simulink model "observer"  (R2023b)
settings: Solver=VariableStepAuto  StartTime=0.0  StopTime=10.0  FixedStep=0.0066666666666666671  MaxStep=0.1e-3
undefined symbols (not defined in the file or in its folder): A_obs, AMPLITUDE, B_obs, C_obs, D_obs, FREQUENCY
settings Model: Creator=gosmann  LastModifiedBy=gosmann
settings SolverCC: MaxConsecutiveMinStep=100

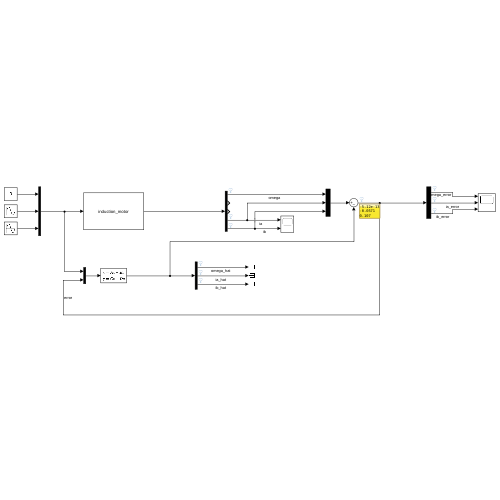
[thumbnail: Simulink's stored preview of the top-level diagram]
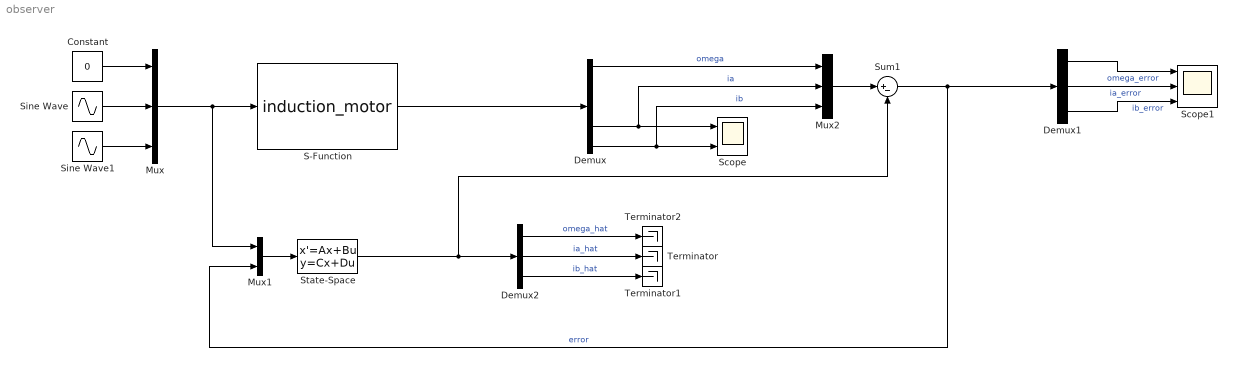
== system observer ==
  Constant : Constant  Value=0
  Demux : Demux  Outputs=5
  Demux1 : Demux  Outputs=3
  Demux2 : Demux  Outputs=3
  Mux : Mux  Inputs=3
  Mux1 : Mux  Inputs=2
  Mux2 : Mux  Inputs=3
  S-Function : S-Function  FunctionName=induction_motor  Parameters=parameters  SFunctionDeploymentMode=off  EnableBusSupport=off
  Scope : Scope  NumInputPorts=2
  Scope1 : Scope  NumInputPorts=3
  Sine Wave : Sin  Amplitude=AMPLITUDE  Frequency=FREQUENCY  SampleTime=0
  Sine Wave1 : Sin  Amplitude=AMPLITUDE  Frequency=FREQUENCY  Phase=0-(pi/180)*90  SampleTime=0
  State-Space : StateSpace  A=A_obs  B=B_obs  C=C_obs  D=D_obs  InitialCondition=[ 0 0 0 0 0 ]
  Sum1 : Sum  Inputs=|+-
  Terminator : Terminator
  Terminator1 : Terminator
  Terminator2 : Terminator
  wires:
  S-Function/1 -> Demux/1
  Mux/1 -> Mux1/1, S-Function/1
  Sine Wave1/1 -> Mux/3
  Sine Wave/1 -> Mux/2
  Constant/1 -> Mux/1
  Demux/4 -> Mux2/2, Scope/1  "ia"
  Demux/5 -> Mux2/3, Scope/2  "ib"
  Mux1/1 -> State-Space/1
  Demux/1 -> Mux2/1  "omega"
  Mux2/1 -> Sum1/1
  State-Space/1 -> Demux2/1, Sum1/2
  Sum1/1 -> Mux1/2, Demux1/1  "error"
  Demux1/1 -> Scope1/1  "omega_error"
  Demux1/2 -> Scope1/2  "ia_error"
  Demux1/3 -> Scope1/3  "ib_error"
  Demux2/2 -> Terminator/1  "ia_hat"
  Demux2/1 -> Terminator2/1  "omega_hat"
  Demux2/3 -> Terminator1/1  "ib_hat"
